simulink model "PropuestaControl"  (R2022b)
settings: Solver=ode4  StartTime=0.0  StopTime=60  FixedStep=0.001  RelTol=1e-3
undefined symbols (not defined in the file): A, B, k, kd, nodeControl, nodeDisturbe, Psi1, Psi2, V0, W1, W2
settings Model: Creator=raul  LastModifiedBy=raul

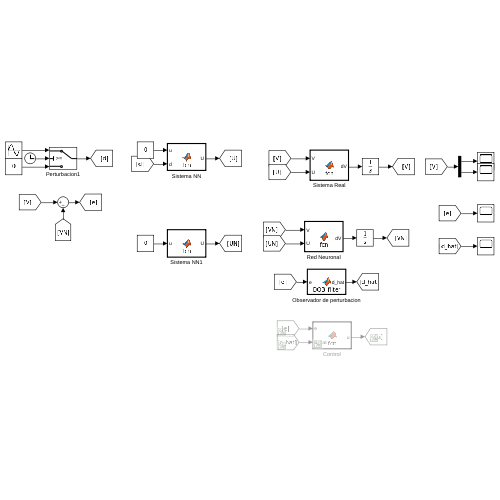
[thumbnail: Simulink's stored preview of the top-level diagram]
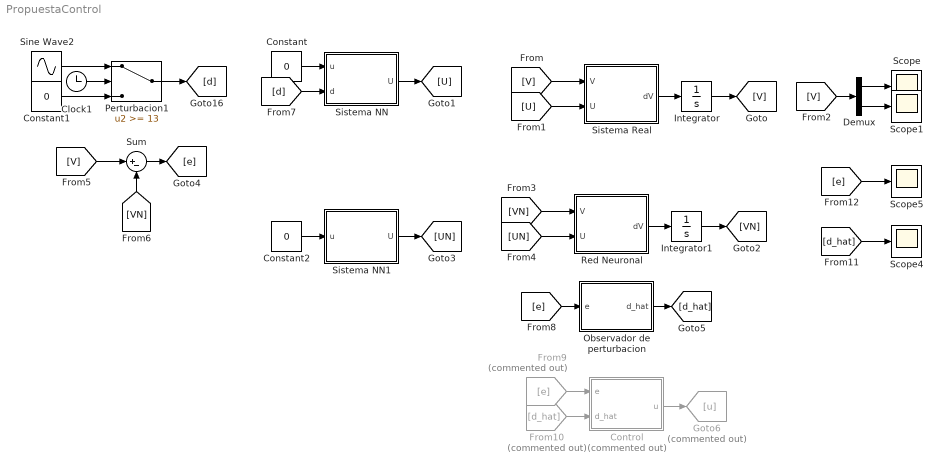
== system PropuestaControl ==
  Clock1 : Clock
  Constant : Constant  Value=0
  Constant1 : Constant  Value=0
  Constant2 : Constant  Value=0
  Control : MATLAB Function  Commented=on  TreatAsAtomicUnit=on
  Demux : Demux  Outputs=2
  From10 : From  Commented=on  GotoTag=d_hat
  From9 : From  Commented=on  GotoTag=e
  Goto6 : Goto  Commented=on  GotoTag=u
  Integrator : Integrator  InitialCondition=V0
  Integrator1 : Integrator  InitialCondition=V0
  Observador de perturbacion : MATLAB Function  TreatAsAtomicUnit=on
  Perturbacion1 : Switch  Threshold=13  SaturateOnIntegerOverflow=off  InputSameDT=off
  Red Neuronal : MATLAB Function  TreatAsAtomicUnit=on
  Scope{,1,4..5} (4 alike) : Scope
  Sine Wave2 : Sin  Frequency=10  SampleTime=0
  Sistema NN : MATLAB Function  TreatAsAtomicUnit=on
  Sistema NN1 : MATLAB Function  TreatAsAtomicUnit=on
  Sistema Real : MATLAB Function  TreatAsAtomicUnit=on
  Sum : Sum  Inputs=|+-
  wires:
  Sistema Real/1(dV) -> Integrator/1
  Integrator/1 -> [V]
  [V] -> Sistema Real/1(V)
  [U] -> Sistema Real/2(U)
  Sistema NN/1(U) -> [U]
  [V] -> Demux/1
  Demux/1 -> Scope/1
  Demux/2 -> Scope1/1
  [VN] -> Red Neuronal/1(V)
  Red Neuronal/1(dV) -> Integrator1/1
  Integrator1/1 -> [VN]
  [V] -> Sum/1
  [VN] -> Sum/2
  Perturbacion1/1 -> [d]
  Sine Wave2/1 -> Perturbacion1/1
  Clock1/1 -> Perturbacion1/2
  Constant1/1 -> Perturbacion1/3
  [d] -> Sistema NN/2(d)
  Constant/1 -> Sistema NN/1(u)
  [UN] -> Red Neuronal/2(U)
  Constant2/1 -> Sistema NN1/1(u)
  Sistema NN1/1(U) -> [UN]
  Sum/1 -> [e]
  [e] -> Observador de perturbacion/1(e)
  From9/1 -> Control/1(e)
  From10/1 -> Control/2(d_hat)
  Observador de perturbacion/1(d_hat) -> [d_hat]
  Control/1(u) -> Goto6/1
  [d_hat] -> Scope4/1
  [e] -> Scope5/1

== matlab function PropuestaControl/Sistema NN ==
  data: U output; u input; d input; nodeControl parameter; nodeDisturbe parameter
function U = fcn(u,d, nodeControl, nodeDisturbe)%add Bw,w

U=zeros(20,1);
U(nodeDisturbe,1)=d;
U(nodeControl,1)=u;

== matlab function PropuestaControl/Sistema Real ==
  data: V input; U input; dV output; W1 parameter; W2 parameter; Psi1 parameter; Psi2 parameter; B parameter; A parameter
function dV  = fcn(V, U, W1, W2, Psi1, Psi2, B, A)

dV=A*V+B*(W1*sigmoid(Psi1,V)+W2*phi_sigmoid(Psi2,V)*U);


function s = sigmoid(b,x)
   s = 1./(1+exp(-b*x)); 
end



function phi = phi_sigmoid(bp, xp)
    % Comprueba que b y x tengan las dimensiones adecuadas
    [rows_b, cols_b] = size(bp);
%     [rows_x, cols_x] = size(xp);

    % Inicializa la matriz de salida
    phi = zeros(rows_b, rows_b); % Matriz de 20x20

    % Calcula la sigmoide combinando cada fila de b con el vector x
    for i = 1:rows_b
        phi(i, :) = 1 ./ (1 + exp(-bp(i, :) * xp)); % Producto y sigmoide
    end
end



end

== matlab function PropuestaControl/Red Neuronal ==
  data: V input; U input; dV output; W1 parameter; W2 parameter; Psi1 parameter; Psi2 parameter; B parameter; A parameter
function dV  = fcn(V, U, W1, W2, Psi1, Psi2, B, A)

dV=A*V+B*(W1*sigmoid(Psi1,V)+W2*phi_sigmoid(Psi2,V)*U);


function s = sigmoid(b,x)
   s = 1./(1+exp(-b*x)); 
end



function phi = phi_sigmoid(bp, xp)
    % Comprueba que b y x tengan las dimensiones adecuadas
    [rows_b, cols_b] = size(bp);
%     [rows_x, cols_x] = size(xp);

    % Inicializa la matriz de salida
    phi = zeros(rows_b, rows_b); % Matriz de 20x20

    % Calcula la sigmoide combinando cada fila de b con el vector x
    for i = 1:rows_b
        phi(i, :) = 1 ./ (1 + exp(-bp(i, :) * xp)); % Producto y sigmoide
    end
end



end

== matlab function PropuestaControl/Observador de perturbacion ==
  settings: updateMethod=DISCRETE
  data: e input; d_hat output
function d_hat = DOB_filter(e)
% Filtro Butterworth de 2do orden (15 Hz)
persistent b a z
if isempty(b)
    Fs = 1000;       % Frecuencia de muestreo
    fc = 15;         % Frecuencia de corte
    [b, a] = butter(2, fc/(Fs/2)); % Coeficientes
    z = zeros(2, 1); % Estados del filtro (condiciones iniciales)
end

% Aplica el filtro (formato Direct Form II)
[d_hat, z] = filter(b, a, e, z);
end

== matlab function PropuestaControl/Sistema NN1 ==
  data: U output; u input; nodeControl parameter
function U = fcn(u, nodeControl)%add Bw,w

U=zeros(20,1);
U(nodeControl,1)=u;

== matlab function PropuestaControl/Control ==
  data: e input; u output; d_hat input; k parameter; kd parameter
function u = fcn(e,d_hat,k, kd)

u=-k*e-kd*d_hat;
